simulink model "testModel"  (R2020a)
settings: Solver=VariableStepAuto  StartTime=0.0  StopTime=10.0  RelTol=1e-3  EnableMultiTasking=on
values from neighbouring files (symbols this model uses):
  mv0 = u0(1)    [runSim.m]
  Ts = 0.001    [runSim.m]
  x0 = [0;0]    [runSim.m]
libraries: mympclib x1
settings Model: ExtModeTrigDuration=2  Creator=kohei  LastModifiedBy=kohei
settings OptimizationCC: DefaultParameterBehavior=Inlined  EnhancedBackFolding=on  PassReuseOutputArgsAs=Individual arguments  MaxStackSize=64  OptimizeBlockOrder=speed  DifferentSizesBufferReuse=on  OptimizationCustomize=off  EfficientTunableParamExpr=on
settings DebuggingCC: ParameterTunabilityLossMsg=error
settings HardwareCC: ProdBitPerInt=16  ProdBitPerPointer=16  ProdBitPerSizeT=16  ProdBitPerPtrDiffT=16  ProdLargestAtomicFloat=None  ProdWordSize=8  ProdHWDeviceType=Atmel->AVR
settings SFSimCC: MATLABDynamicMemAlloc=off  CustomCodeUndefinedFunction=UseInterfaceOnly
settings RTWCC: SystemTargetFile=ert.tlc  TemplateMakefile=ert_default_tmf  GenerateReport=on  Toolchain=Arduino AVR  BuildConfiguration=Faster Runs  IncludeHyperlinkInReport=on  LaunchReport=on  GenerateTraceInfo=on  GenerateTraceReport=on  GenerateTraceReportSl=on  GenerateTraceReportSf=on  GenerateTraceReportEml=on
settings CodeAppCC: ForceParamTrailComments=on  IgnoreCustomStorageClasses=off  OperatorAnnotations=on  SimulinkDataObjDesc=on  SFDataObjDesc=on  InsertBlockDesc=on
settings ERTTargetCC: SupportContinuousTime=on  SupportVariableSizeSignals=on  ExtModeStaticAllocSize=2048  ERTCustomFileTemplate=example_file_process.tlc

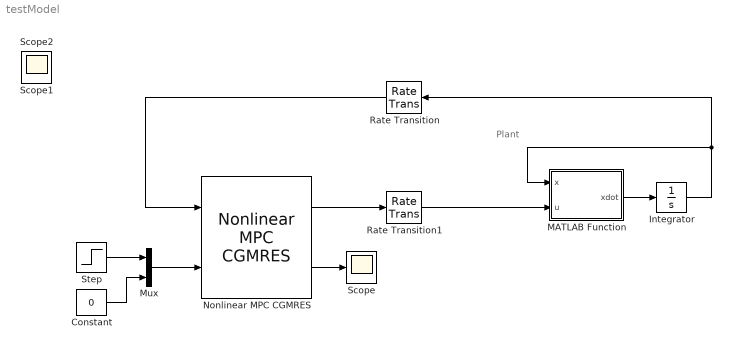
== system testModel ==
  note: Plant
  Constant : Constant  Value=0  SampleTime=Ts
  Integrator : Integrator  InitialCondition=x0
  MATLAB Function : MATLAB Function  TreatAsAtomicUnit=on
  Mux : Mux  Inputs=2
  Nonlinear MPC CGMRES : mympclib/Nonlinear MPC CGMRES  params=params  nx=2  nmv=1  ns=1  nL=1  Ts=Ts  enableDist=off  nd=0  enableStatus=on
      settings: SourceProductName=My MPC Library
  Rate Transition : RateTransition  InitialCondition=x0
  Rate Transition1 : RateTransition  InitialCondition=mv0
  Scope : Scope
  Step : Step  After=2  SampleTime=Ts
  Scope1 : Scope
  Scope2 : Scope
  wires:
  Nonlinear MPC CGMRES/1 -> Rate Transition1/1
  Nonlinear MPC CGMRES/2 -> Scope/1
  MATLAB Function/1(xdot) -> Integrator/1
  Integrator/1 -> MATLAB Function/1(x), Rate Transition/1
  Mux/1 -> Nonlinear MPC CGMRES/2
  Step/1 -> Mux/1
  Constant/1 -> Mux/2
  Rate Transition1/1 -> MATLAB Function/2(u)
  Rate Transition/1 -> Nonlinear MPC CGMRES/1

== matlab function testModel/MATLAB Function ==
  data: x input; u input; xdot output
function xdot = fcn(x,u)
xdot = plant(x,u);
end
